simulink model "simulinkmodel"  (R2022a)
settings: Solver=VariableStepAuto  StartTime=0.0  StopTime=10.0  RelTol=1e-3
undefined symbols (not defined in the file or in its folder): A, Ad_hat_100, B, Bd_hat_100, K_d
settings Model: Creator=user  LastModifiedBy=user

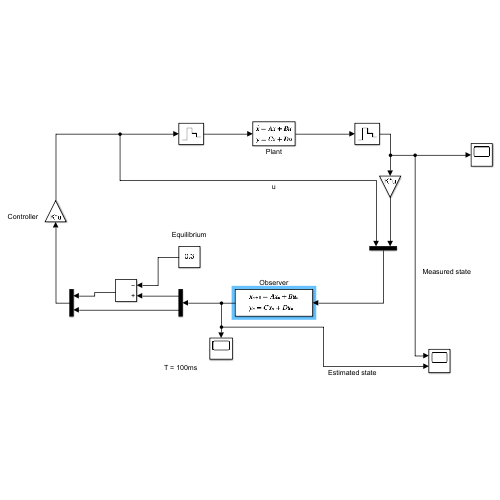
[thumbnail: Simulink's stored preview of the top-level diagram]
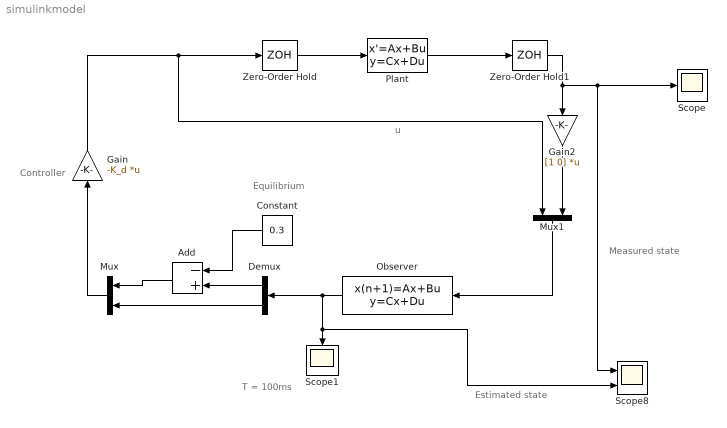
== system simulinkmodel ==
  note: Measured state
  note: Equilibrium
  note: Controller
  note: u
  note: T = 100ms
  note: Estimated state
  Add : Sum  Inputs=-+
  Constant : Constant  Value=0.3
  Demux : Demux  Outputs=2
  Gain : Gain  Gain=-K_d  Multiplication=Matrix(K*u)
  Gain2 : Gain  Gain=[1 0]  Multiplication=Matrix(K*u)
  Mux : Mux  Inputs=2
  Mux1 : Mux  Inputs=2
  Observer : DiscreteStateSpace  A=Ad_hat_100  B=Bd_hat_100  C=eye(2)  D=[0 0;0 0]  SampleTime=0.1
  Plant : StateSpace  A=A  B=B  C=eye(2)  D=[0;0]  InitialCondition=0
  Scope : Scope
  Scope1 : Scope
  Scope8 : Scope  NumInputPorts=2
  Zero-Order Hold : ZeroOrderHold  SampleTime=0.1
  Zero-Order Hold1 : ZeroOrderHold  SampleTime=0.1
  wires:
  Plant/1 -> Zero-Order Hold1/1
  Gain2/1 -> Mux1/2
  Mux/1 -> Gain/1
  Observer/1 -> Demux/1, Scope8/2, Scope1/1
  Add/1 -> Mux/1
  Zero-Order Hold1/1 -> Scope8/1, Scope/1, Gain2/1
  Constant/1 -> Add/1
  Mux1/1 -> Observer/1
  Gain/1 -> Mux1/1, Zero-Order Hold/1
  Demux/2 -> Mux/2
  Demux/1 -> Add/2
  Zero-Order Hold/1 -> Plant/1
